simulink model "model_validation_Va_OL"  (R2023b)
settings: Solver=VariableStepAuto  StartTime=0.0  StopTime=30.0  RelTol=1e-3
values from neighbouring files (symbols this model uses):
  A = double(A)    [consistent.m]    (also in dyn_model_mark.m)
  B = double(B)    [consistent.m]    (also in dyn_model_mark.m)
  C = [1 0 0 0 ... (first row only)    [consistent.m]    (also in dyn_model_mark.m)
  D = [0 ... (first row only)    [consistent.m]    (also in dyn_model_mark.m)
  g0 = 9.81    [consistent.m]    (also in dyn_model_mark.m)
  Ip = (mp*Lp^2)/12    (= 3.3282e-05)    [consistent.m]    (also in dyn_model_mark.m = 8.3205e-06)
  Ir = (mr*Lr^2)/12    (= 5.71979166667e-05)    [consistent.m]    (also in dyn_model_mark.m = 1.42994791667e-05)
  K = place(A,B,P)    [consistent.m]    (also in dyn_model_mark.m)
  La = 1.16e-3    (= 0.00116)    [consistent.m]    (also in dyn_model_mark.m)
  Lp = 0.129    [consistent.m]    (also in dyn_model_mark.m = 0.0645)
  Lr = 0.085    [consistent.m]    (also in dyn_model_mark.m)
  mp = 0.024    [consistent.m]    (also in dyn_model_mark.m)
  mr = 0.095    [consistent.m]    (also in dyn_model_mark.m)
  phi_dot_init = 0    [consistent.m]
  phi_init = 0    [consistent.m]
  R_tilde = zeros(2,2)    [consistent.m]
  Ra = 8.4    [consistent.m]    (also in dyn_model_mark.m)
  theta_dot_init = 0    [consistent.m]
  theta_init = 0    [consistent.m]
undefined symbols (not defined in the file or in its folder): alfa, beta, Continuous, dist, Ir_tot, Ld, rot_pend, Time
libraries: simulink_extras x7, ctrlSharedLib x1
settings Model: PacingRate=112  Creator=Mark  LastModifiedBy=Mark

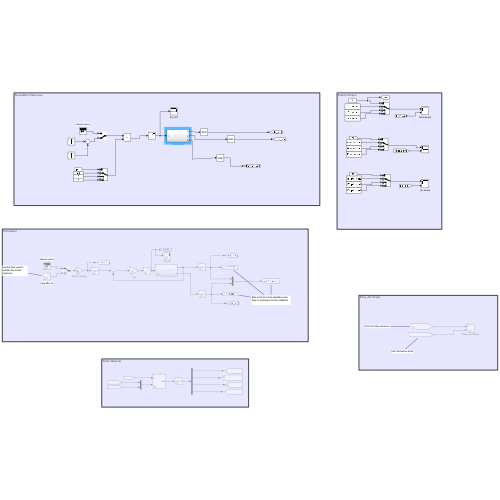
[thumbnail: Simulink's stored preview of the top-level diagram]
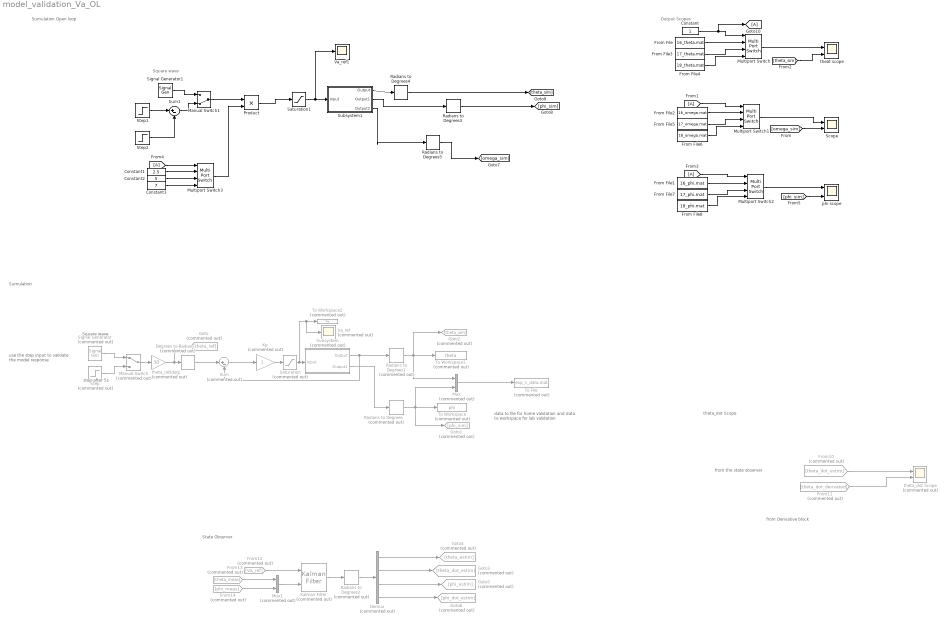
== system model_validation_Va_OL ==
  note: State Observer
  note: Sumulation
  note: theta_dot Scope
  note: from Derivative block
  note: from the state observer
  note: Output Scopes
  note: use the step input to validate the model response
  note: data to file for home validation and data to workspace for lab validation
  note: step after 5s
  note: Square wave
  note: Square wave
  note: Sumulation Open loop
  Constant : Constant
  Constant1 : Constant  Value=2.5
  Constant2 : Constant  Value=5
  Constant3 : Constant  Value=7
  Degrees to Radians : simulink_extras/Transformations/Degrees to Radians  Commented=on
  Demux : Demux  Commented=on
  From File : FromFile  FileName=16_theta.mat  SampleTime=0
  From File1 : FromFile  FileName=16_phi.mat  SampleTime=0
  From File2 : FromFile  FileName=16_omega.mat  SampleTime=0
  From File3 : FromFile  FileName=17_theta.mat  SampleTime=0
  From File4 : FromFile  FileName=18_theta.mat  SampleTime=0
  From File5 : FromFile  FileName=17_omega.mat  SampleTime=0
  From File6 : FromFile  FileName=18_omega.mat  SampleTime=0
  From File7 : FromFile  FileName=17_phi.mat  SampleTime=0
  From File8 : FromFile  FileName=18_phi.mat  SampleTime=0
  From1 : From
  From10 : From  Commented=on  GotoTag=theta_dot_estim
  From11 : From  Commented=on  GotoTag=theta_dot_derivated
  From12 : From  Commented=on  GotoTag=Va_ref
  From13 : From  Commented=on  GotoTag=theta_meas
  From14 : From  Commented=on  GotoTag=phi_meas
  From3 : From
  From4 : From
  Goto : Goto  Commented=on  GotoTag=theta_ref
  Goto1 : Goto  Commented=on  GotoTag=phi_sim
  Goto10 : Goto
  Goto2 : Goto  Commented=on  GotoTag=theta_sim
  Goto3 : Goto  Commented=on  GotoTag=theta_dot_estim
  Goto4 : Goto  Commented=on  GotoTag=theta_estim
  Goto5 : Goto  Commented=on  GotoTag=phi_estim
  Goto6 : Goto  Commented=on  GotoTag=phi_dot_estim
  Kalman Filter : ctrlSharedLib/Kalman Filter  Commented=on  TimeDomain=Continuous-Time  UseCurrentEstimator=on  ModelSource=Individual A, B, C, D matrices  ModelSourceVariable=ss(0.95,1,1,0,1)  A=A  B=B  C=C  D=D  NumberOfStates=1  NumberOfInputs=1  NumberOfOutputs=1  InitialEstimateSource=Dialog  X0=[0 0 pi 0]  P0=10  UseK=off  UseGH=off  NumberOfProcessNoiseInputs=1  G=1  TimeInvariantG=on  H=0  TimeInvariantH=on  Q=Q_tilde  TimeInvariantQ=on  R=R_tilde  TimeInvariantR=on  N=0  TimeInvariantN=on  AddInputPort=on  AddEnablePort=off  OutputEstimatedY=off  OutputP=off  Ts=-1
  Kp : Gain  Commented=on
  Manual Switch : ManualSwitch  Commented=on
  Manual Switch1 : ManualSwitch  CurrentSetting=0
  Multiport Switch{,1..3} (4 alike) : MultiPortSwitch  SaturateOnIntegerOverflow=off  InputSameDT=off
  Mux : Mux  Commented=on  Inputs=2
  Mux1 : Mux  Commented=on  Inputs=2
  Product : Product
  Radians to Degrees : simulink_extras/Transformations/Radians to Degrees  Commented=on
  Radians to Degrees1 : simulink_extras/Transformations/Radians to Degrees  Commented=on
  Radians to Degrees2 : simulink_extras/Transformations/Radians to Degrees  Commented=on
  Radians to Degrees3 : simulink_extras/Transformations/Radians to Degrees
  Radians to Degrees4 : simulink_extras/Transformations/Radians to Degrees
  Radians to Degrees5 : simulink_extras/Transformations/Radians to Degrees
  Saturation : Saturate  Commented=on  UpperLimit=10  LowerLimit=-10
  Saturation1 : Saturate  UpperLimit=10  LowerLimit=-10
  Scope : Scope  NumInputPorts=2
  Signal Generator : SignalGenerator  Commented=on  WaveForm=square  Frequency=0.05
  Signal Generator1 : SignalGenerator  WaveForm=square  Frequency=0.1
  Step : Step  Commented=on  Time=5  SampleTime=0
  Step1 : Step  SampleTime=0
  Step2 : Step  Time=1.05  SampleTime=0
  Subsystem : Subsystem  Commented=on
  Subsystem1 : Subsystem
  Sum : Sum  Commented=on  Inputs=|+-
  Sum1 : Sum  Inputs=|+-
  To File : ToFile  Commented=on  Filename=exp_1_data.mat  MatrixName=angle
  To Workspace : ToWorkspace  Commented=on  VariableName=phi  SampleTime=-1
  To Workspace1 : ToWorkspace  Commented=on  VariableName=theta  SampleTime=-1
  To Workspace2 : ToWorkspace  Commented=on  VariableName=Va  SampleTime=-1
  Va_ref : Scope  Commented=on
  Va_ref1 : Scope
  phi scope : Scope  NumInputPorts=2
  theat scope : Scope  NumInputPorts=2
  theta_dot Scope : Scope  Commented=on  NumInputPorts=2
  theta_ref(deg) : Gain  Commented=on  Gain=30
  wires:
  Mux/1 -> To File/1
  Kp/1 -> Saturation/1
  Saturation/1 -> Va_ref/1, To Workspace2/1, Subsystem/1(Input)
  Step/1 -> Manual Switch/2
  Signal Generator/1 -> Manual Switch/1
  Radians to Degrees1/1 -> Goto2/1, To Workspace1/1, Mux/1
  Degrees to Radians/1 -> Sum/1
  Subsystem/2(Output1) -> Radians to Degrees/1
  Radians to Degrees/1 -> Mux/2, To Workspace/1, Goto1/1
  Sum/1 -> Kp/1
  Manual Switch/1 -> theta_ref(deg)/1
  [theta_sim] -> theat scope/2
  From File/1 -> Multiport Switch/2
  [phi_sim] -> phi scope/2
  From10/1 -> theta_dot Scope/1
  From11/1 -> theta_dot Scope/2
  Radians to Degrees2/1 -> Demux/1
  Kalman Filter/1 -> Radians to Degrees2/1
  Mux1/1 -> Kalman Filter/2
  From12/1 -> Kalman Filter/1
  From13/1 -> Mux1/1
  From14/1 -> Mux1/2
  Demux/2 -> Goto3/1
  Demux/1 -> Goto4/1
  Demux/3 -> Goto5/1
  Demux/4 -> Goto6/1
  theta_ref(deg)/1 -> Goto/1, Degrees to Radians/1
  Subsystem/1(Output) -> Sum/2, Radians to Degrees1/1
  Product/1 -> Saturation1/1
  Subsystem1/2(Output1) -> Radians to Degrees3/1
  Radians to Degrees3/1 -> [phi_sim]
  Manual Switch1/1 -> Product/1
  Saturation1/1 -> Va_ref1/1, Subsystem1/1(Input)
  Step1/1 -> Sum1/1
  Radians to Degrees4/1 -> [theta_sim]
  Signal Generator1/1 -> Manual Switch1/1
  Sum1/1 -> Manual Switch1/2
  Step2/1 -> Sum1/2
  From File1/1 -> Multiport Switch2/2
  Subsystem1/1(Output) -> Radians to Degrees4/1
  From File2/1 -> Multiport Switch1/2
  Radians to Degrees5/1 -> [omega_sim]
  Subsystem1/3(Output2) -> Radians to Degrees5/1
  [omega_sim] -> Scope/2
  Multiport Switch/1 -> theat scope/1
  Constant/1 -> Goto10/1, Multiport Switch/1
  From File3/1 -> Multiport Switch/3
  From File4/1 -> Multiport Switch/4
  Multiport Switch1/1 -> Scope/1
  From File5/1 -> Multiport Switch1/3
  From File6/1 -> Multiport Switch1/4
  From1/1 -> Multiport Switch1/1
  From3/1 -> Multiport Switch2/1
  From File7/1 -> Multiport Switch2/3
  From File8/1 -> Multiport Switch2/4
  Multiport Switch2/1 -> phi scope/1
  Multiport Switch3/1 -> Product/2
  From4/1 -> Multiport Switch3/1
  Constant1/1 -> Multiport Switch3/2
  Constant2/1 -> Multiport Switch3/3
  Constant3/1 -> Multiport Switch3/4

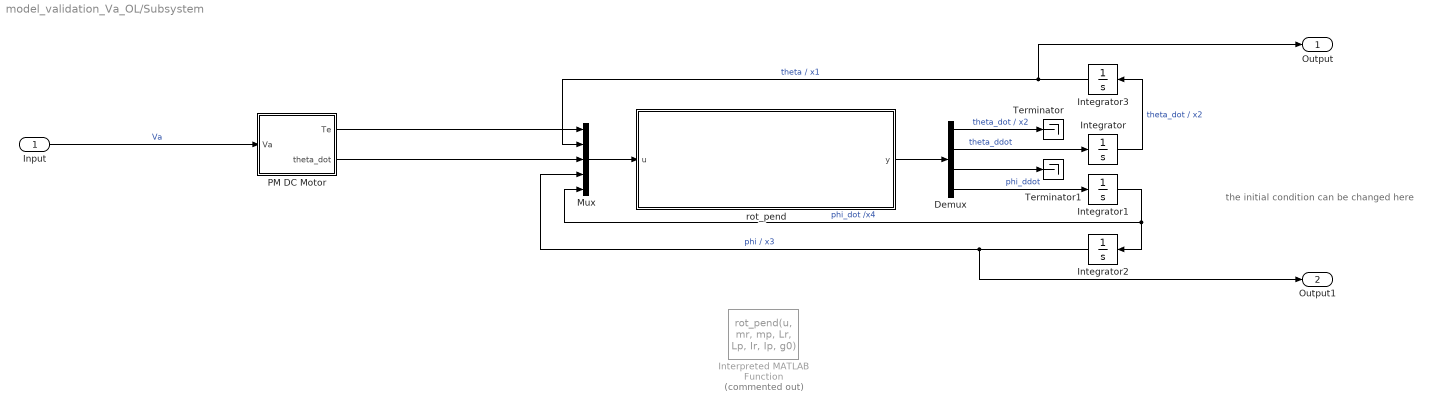
== system model_validation_Va_OL/Subsystem ==
  note: the initial condition can be changed here
  Input : Inport
  Demux : Demux
  Integrator : Integrator  InitialCondition=theta_dot_init
  Integrator1 : Integrator  InitialCondition=phi_dot_init
  Integrator2 : Integrator  InitialCondition=phi_init
  Integrator3 : Integrator  InitialCondition=theta_init
  Interpreted MATLAB Function : MATLABFcn  Commented=on  MATLABFcn=rot_pend(u, mr, mp, Lr, Lp, Ir, Ip, g0)  OutputDimensions=4  OutputSignalType=real
  Mux : Mux  Inputs=5
  PM DC Motor : Subsystem
  Terminator : Terminator
  Terminator1 : Terminator
  rot_pend : Subsystem
  Output : Outport
  Output1 : Outport  Port=2
  wires:
  Integrator2/1 -> Output1/1, Mux/4  "phi / x3"
  Integrator/1 -> Integrator3/1  "theta_dot / x2"
  Mux/1 -> rot_pend/1(u)
  rot_pend/1(y) -> Demux/1
  Integrator1/1 -> Mux/5, Integrator2/1  "phi_dot /x4"
  Integrator3/1 -> Mux/2, Output/1  "theta / x1"
  Demux/4 -> Integrator1/1  "phi_ddot"
  Demux/2 -> Integrator/1  "theta_ddot"
  Demux/1 -> Terminator/1  "theta_dot / x2"
  Demux/3 -> Terminator1/1
  Input/1 -> PM DC Motor/1(Va)  "Va"
  PM DC Motor/1(Te) -> Mux/1
  PM DC Motor/2(theta_dot) -> Mux/3

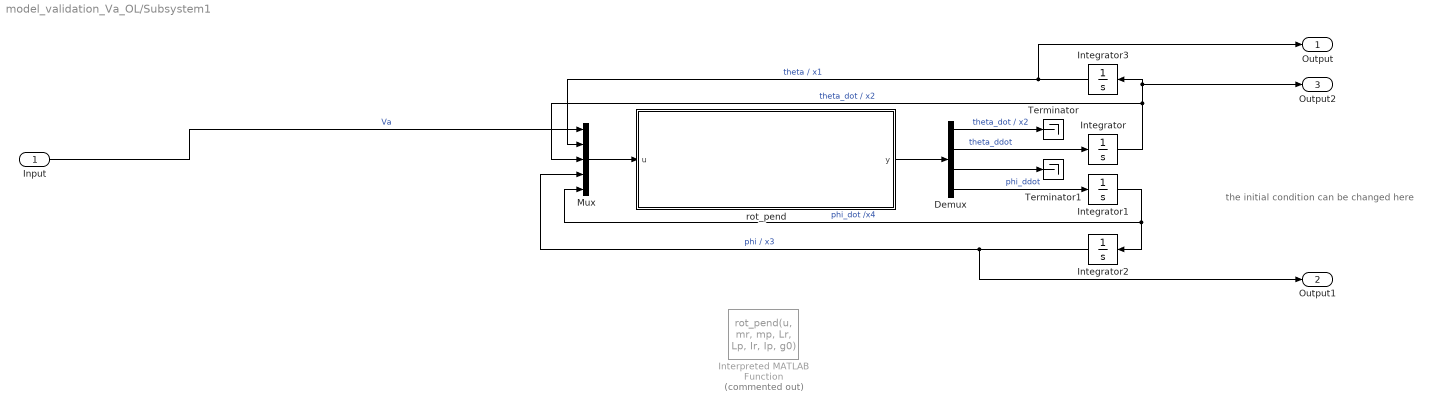
== system model_validation_Va_OL/Subsystem1 ==
  note: the initial condition can be changed here
  Input : Inport
  Demux : Demux
  Integrator : Integrator  InitialCondition=theta_dot_init
  Integrator1 : Integrator  InitialCondition=phi_dot_init
  Integrator2 : Integrator  InitialCondition=phi_init
  Integrator3 : Integrator  InitialCondition=theta_init
  Interpreted MATLAB Function : MATLABFcn  Commented=on  MATLABFcn=rot_pend(u, mr, mp, Lr, Lp, Ir, Ip, g0)  OutputDimensions=4  OutputSignalType=real
  Mux : Mux  Inputs=5
  Terminator : Terminator
  Terminator1 : Terminator
  rot_pend : Subsystem
  Output : Outport
  Output1 : Outport  Port=2
  Output2 : Outport  Port=3
  wires:
  Integrator2/1 -> Output1/1, Mux/4  "phi / x3"
  Integrator/1 -> Output2/1, Integrator3/1, Mux/3  "theta_dot / x2"
  Mux/1 -> rot_pend/1(u)
  rot_pend/1(y) -> Demux/1
  Integrator1/1 -> Mux/5, Integrator2/1  "phi_dot /x4"
  Integrator3/1 -> Mux/2, Output/1  "theta / x1"
  Demux/4 -> Integrator1/1  "phi_ddot"
  Demux/2 -> Integrator/1  "theta_ddot"
  Demux/1 -> Terminator/1  "theta_dot / x2"
  Demux/3 -> Terminator1/1
  Input/1 -> Mux/1  "Va"

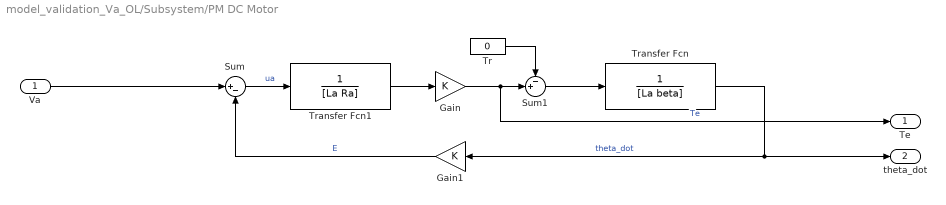
== system model_validation_Va_OL/Subsystem/PM DC Motor ==
  Va : Inport
  Gain : Gain  Gain=K
  Gain1 : Gain  Gain=K
  Sum : Sum  Inputs=|+-
  Sum1 : Sum  Inputs=-+|
  Tr : Constant  Value=0
  Transfer Fcn : TransferFcn  Denominator=[La beta]
  Transfer Fcn1 : TransferFcn  Denominator=[La Ra]
  Te : Outport
  theta_dot : Outport  Port=2
  wires:
  Sum1/1 -> Transfer Fcn/1
  Gain/1 -> Te/1, Sum1/2  "Te"
  Transfer Fcn/1 -> Gain1/1, theta_dot/1  "theta_dot"
  Gain1/1 -> Sum/2  "E"
  Va/1 -> Sum/1
  Sum/1 -> Transfer Fcn1/1  "ua"
  Tr/1 -> Sum1/1
  Transfer Fcn1/1 -> Gain/1

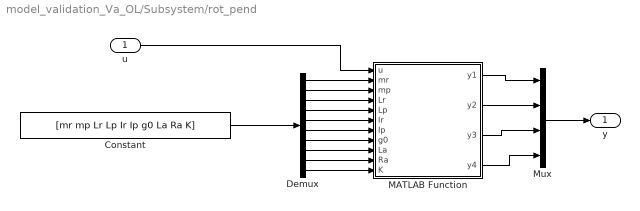
== system model_validation_Va_OL/Subsystem/rot_pend ==
  u : Inport
  Constant : Constant  Value=[mr mp Lr Lp Ir Ip g0 La Ra K]  VectorParams1D=off
  Demux : Demux  Outputs=10
  MATLAB Function : MATLAB Function  TreatAsAtomicUnit=on
  Mux : Mux
  y : Outport
  wires:
  Demux/3 -> MATLAB Function/4(Lr)
  Demux/5 -> MATLAB Function/6(Ir)
  Demux/4 -> MATLAB Function/5(Lp)
  Demux/7 -> MATLAB Function/8(g0)
  Demux/2 -> MATLAB Function/3(mp)
  Demux/6 -> MATLAB Function/7(Ip)
  Demux/1 -> MATLAB Function/2(mr)
  u/1 -> MATLAB Function/1(u)
  Constant/1 -> Demux/1
  MATLAB Function/1(y1) -> Mux/1
  MATLAB Function/2(y2) -> Mux/2
  MATLAB Function/3(y3) -> Mux/3
  MATLAB Function/4(y4) -> Mux/4
  Mux/1 -> y/1
  Demux/8 -> MATLAB Function/9(La)
  Demux/9 -> MATLAB Function/10(Ra)
  Demux/10 -> MATLAB Function/11(K)

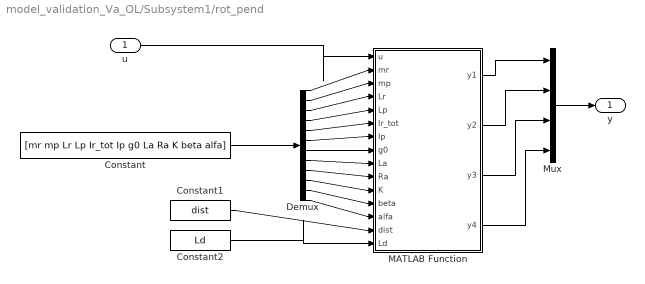
== system model_validation_Va_OL/Subsystem1/rot_pend ==
  u : Inport
  Constant : Constant  Value=[mr mp Lr Lp Ir_tot Ip g0 La Ra K beta alfa]  VectorParams1D=off
  Constant1 : Constant  Value=dist
  Constant2 : Constant  Value=Ld
  Demux : Demux  Outputs=12
  MATLAB Function : MATLAB Function  TreatAsAtomicUnit=on
  Mux : Mux
  y : Outport
  wires:
  Demux/3 -> MATLAB Function/4(Lr)
  Demux/5 -> MATLAB Function/6(Ir_tot)
  Demux/4 -> MATLAB Function/5(Lp)
  Demux/7 -> MATLAB Function/8(g0)
  Demux/2 -> MATLAB Function/3(mp)
  Demux/6 -> MATLAB Function/7(Ip)
  Demux/1 -> MATLAB Function/2(mr)
  u/1 -> MATLAB Function/1(u)
  Constant/1 -> Demux/1
  MATLAB Function/1(y1) -> Mux/1
  MATLAB Function/2(y2) -> Mux/2
  MATLAB Function/3(y3) -> Mux/3
  MATLAB Function/4(y4) -> Mux/4
  Mux/1 -> y/1
  Demux/8 -> MATLAB Function/9(La)
  Demux/9 -> MATLAB Function/10(Ra)
  Demux/10 -> MATLAB Function/11(K)
  Demux/11 -> MATLAB Function/12(beta)
  Constant1/1 -> MATLAB Function/14(dist)
  Constant2/1 -> MATLAB Function/15(Ld)
  Demux/12 -> MATLAB Function/13(alfa)

== matlab function model_validation_Va_OL/Subsystem1/rot_pend/MATLAB Function ==
  data: u input; y1 output; mr input; mp input; Lr input; Lp input; Ir_tot input; Ip input; g0 input; La input; Ra input; y2 output; y3 output; y4 output; K input; beta input; alfa input; dist input; Ld input
function [y1,y2,y3,y4] = rot_pend(u, mr, mp, Lr, Lp, Ir_tot, Ip, g0,La, Ra, K, beta,alfa, dist, Ld)
%UNTITLED Summary of this function goes here
%   Detailed explanation goes here
% u(1) = Va
x1 = u(2) ; % theta
x2 = u(3) ; % theta_dot
x3 = u(4) ; % phi
x4 = u(5) ; % phi_dot

H = [(mp*(Lr^2+((Lp/2)^2*(sin(x3))^2)))+Ir_tot            -mp*Lr*Lp*cos(x3)/2;
                     -mp*Lr*Lp*cos(x3)/2                              (mp*(Lp/2)^2)+Ip] ;

Q = [mp*(Lp/2)^2*sin(x3)*cos(x3)*x4+beta                     (mp*(Lp/2)^2*sin(x3)*cos(x3)*x2)-(mp*Lr*(Lp/2)*sin(x3)*x4);
     -mp*(Lp/2)^2*sin(x3)*cos(x3)*x2                                                   alfa                                   ] ;

g = [           0     ;
     mp*g0*(Lp/2)*sin(x3)] ;
%(K*u(1)/Ra)-(K^2*x2/Ra)
tau = [(K/Ra)*(u(1)-(K*x2)) ;
       0 ] ;

if (x1>=0.1745 | x1<=-0.1745)       % 0.08727rad = 5deg
     kt = 0.03 ;                    % 0.1745rad = 10deg
     kc = 10e-3 ;
else                               % 0.349rad = 20deg
    kt = 0 ;
    kc = 3.5e-3 ;
end
% if (x2>=2.618 | x2<=-2.618)       % 3.49rad/s = 200deg/s
%                                 % 2.618rad/s = 150deg/s
%     kc = 10e-3 ;
% else                               
% 
%     kc = 4.8e-3 ;
% end


Tr_theta = ((kt*x1)+(kc*x2))*Ld ;
q_ddot = H\[tau - Q*[x2 x4]' - g - [Tr_theta 0]' ] ;



y1 = x2 ;
y2 = q_ddot(1) ;
y3 = x4 ;
y4 = q_ddot(2) ;


%Ir+mr*(Lr/2)^2)

== matlab function model_validation_Va_OL/Subsystem/rot_pend/MATLAB Function ==
  data: u input; y1 output; mr input; mp input; Lr input; Lp input; Ir input; Ip input; g0 input; La input; Ra input; y2 output; y3 output; y4 output; K input
function [y1,y2,y3,y4] = rot_pend(u, mr, mp, Lr, Lp, Ir, Ip, g0,La, Ra, K)
%UNTITLED Summary of this function goes here
%   Detailed explanation goes here
% u(1) = Te
x1 = u(2) ; % theta
x2 = u(3) ; % theta_dot
x3 = u(4) ; % phi
x4 = u(5) ; % phi_dot

H = [(mp*(Lr^2+((Lp/2)^2*(sin(x3))^2)))+Ir            -mp*Lr*Lp*cos(x3)/2;
                     -mp*Lr*Lp*cos(x3)/2                              (mp*(Lp/2)^2)+Ip] ;

Q = [mp*(Lp/2)^2*sin(x3)*cos(x3)*x4                      (mp*(Lp/2)^2*sin(x3)*cos(x3)*x2)-(mp*Lr*(Lp/2)*sin(x3)*x4);
     -mp*(Lp/2)^2*sin(x3)*cos(x3)*x2                                                   0                                   ] ;

g = [           0     ;
     mp*g0*(Lp/2)*sin(x3)] ;
tau = [u(1);
       0 ] ;

q_ddot = H\[tau - Q*[x2 x4]' - g] ;



y1 = x2 ;
y2 = q_ddot(1) ;
y3 = x4 ;
y4 = q_ddot(2) ;


%Ir+mr*(Lr/2)^2)
